simulink model "baseline_auto_parcel_loading_process"  (R2026a)
settings: Solver=VariableStepAuto  StopTime=500  MaxStep=0.05
libraries: sim3dlib x36
(part 1 of 5)
settings Model: PacingRate=1000  Creator=minho  LastModifiedBy=minho

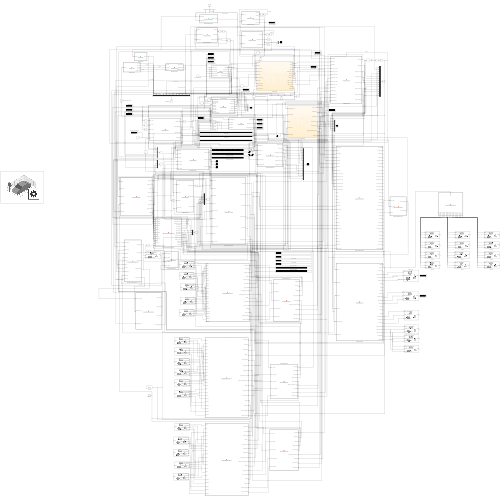
[thumbnail: Simulink's stored preview of the top-level diagram]
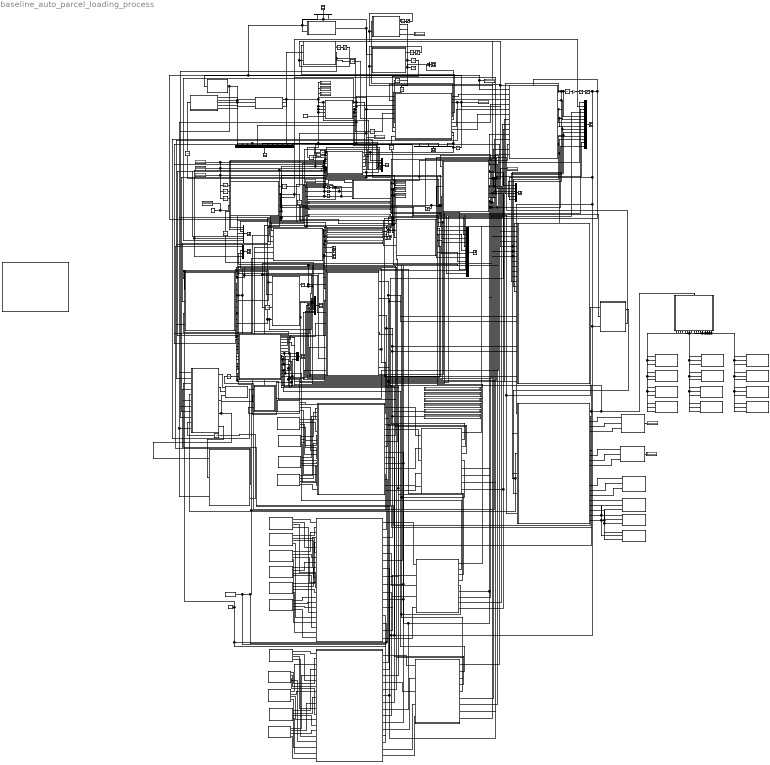
== system baseline_auto_parcel_loading_process ==
  note: floor1_remaining_length
  ArriveDoneDelayToMainController : UnitDelay  SampleTime=0.05
  Belt1_F1 : sim3dlib/Simulation 3D Actor  Priority=1  ActorName=Belt1_F1_Actor  ParentName=Scene Origin  Operation=Create at setup  InitScriptText=|  SampleTime=-1  Translation=[0 0 0]  Rotation=[0 0 0]  Scale=[1 1 1]  InputsText=|  aMode=5  ActorTag=Belt1_F1_Actor  ActorType=Sim3dActor  ID=C
      InitScriptText=|
      | % Reserved keywords:
      | % - Actor : handle to this actor object
      | % - World : handle to the world object
      | 
      | % Examples:
      | 
      | % Create a primitive geometry (optional)
      | createShape(Actor, 'box', [1 1 1]);
      | 
      | % Initialize values (optional)
      | % Actor.Physics = true;
      | Actor.Color = [0.1 0.1 0.1];
      InputsText=|
      | Belt1_F1_Actor.Translation
      | Belt1_F1_Actor.Rotation   
      | Belt1_F1_Actor.Scale
  Belt1_F2 : sim3dlib/Simulation 3D Actor  Priority=1  ActorName=Belt1_F2_Actor  ParentName=Scene Origin  Operation=Create at setup  InitScriptText=|  SampleTime=-1  Translation=[0 0 0]  Rotation=[0 0 0]  Scale=[1 1 1]  InputsText=|  aMode=5  ActorTag=Belt1_F2_Actor  ActorType=Sim3dActor  ID=C
      InitScriptText=|
      | % Reserved keywords:
      | % - Actor : handle to this actor object
      | % - World : handle to the world object
      | createShape(Actor, 'box', [1 1 1]);
      | Actor.Color = [0.1 0.1 0.1];
      | % Examples:
      | 
      | % Create a primitive geometry (optional)
      | % createShape(Actor, 'box', [1 1 1]);
      | 
      | % Initialize values (optional)
      | % Actor.Physics = true;
      | % Actor.Color = [1 0 0];
      InputsText=|
      | Belt1_F2_Actor.Translation
      | Belt1_F2_Actor.Rotation   
      | Belt1_F2_Actor.Scale
  Belt1_F3 : sim3dlib/Simulation 3D Actor  Priority=1  ActorName=Belt1_F3_Actor  ParentName=Scene Origin  Operation=Create at setup  InitScriptText=|  SampleTime=-1  Translation=[0 0 0]  Rotation=[0 0 0]  Scale=[1 1 1]  InputsText=|  aMode=5  ActorTag=Belt1_F3_Actor  ActorType=Sim3dActor  ID=C
      InitScriptText=|
      | % Reserved keywords:
      | % - Actor : handle to this actor object
      | % - World : handle to the world object
      | createShape(Actor, 'box', [1 1 1]);
      | Actor.Color = [0.1 0.1 0.1];
      | % Examples:
      | 
      | % Create a primitive geometry (optional)
      | % createShape(Actor, 'box', [1 1 1]);
      | 
      | % Initialize values (optional)
      | % Actor.Physics = true;
      | % Actor.Color = [1 0 0];
      InputsText=|
      | Belt1_F3_Actor.Translation
      | Belt1_F3_Actor.Rotation   
      | Belt1_F3_Actor.Scale
  Belt2_F1 : sim3dlib/Simulation 3D Actor  Priority=1  ActorName=Belt2_F1_Actor  ParentName=Scene Origin  Operation=Create at setup  InitScriptText=|  SampleTime=-1  Translation=[0 0 0]  Rotation=[0 0 0]  Scale=[1 1 1]  InputsText=|  aMode=5  ActorTag=Belt2_F1_Actor  ActorType=Sim3dActor  ID=C
      InitScriptText=|
      | % Reserved keywords:
      | % - Actor : handle to this actor object
      | % - World : handle to the world object
      | 
      | % Examples:
      | 
      | % Create a primitive geometry (optional)
      | createShape(Actor, 'box', [1 1 1]);
      | 
      | % Initialize values (optional)
      | % Actor.Physics = true;
      | Actor.Color = [0.2 0.2 0.2];
      InputsText=|
      | Belt2_F1_Actor.Translation
      | Belt2_F1_Actor.Rotation   
      | Belt2_F1_Actor.Scale
  Belt2_F2 : sim3dlib/Simulation 3D Actor  Priority=1  ActorName=Belt2_F2_Actor  ParentName=Scene Origin  Operation=Create at setup  InitScriptText=|  SampleTime=-1  Translation=[0 0 0]  Rotation=[0 0 0]  Scale=[1 1 1]  InputsText=|  aMode=5  ActorTag=Belt2_F2_Actor  ActorType=Sim3dActor  ID=C
      InitScriptText=|
      | % Reserved keywords:
      | % - Actor : handle to this actor object
      | % - World : handle to the world object
      | createShape(Actor, 'box', [1 1 1]);
      | Actor.Color = [0.2 0.2 0.2];
      | % Examples:
      | 
      | % Create a primitive geometry (optional)
      | % createShape(Actor, 'box', [1 1 1]);
      | 
      | % Initialize values (optional)
      | % Actor.Physics = true;
      | % Actor.Color = [1 0 0];
      InputsText=|
      | Belt2_F2_Actor.Translation
      | Belt2_F2_Actor.Rotation   
      | Belt2_F2_Actor.Scale
  Belt2_F3 : sim3dlib/Simulation 3D Actor  Priority=1  ActorName=Belt2_F3_Actor  ParentName=Scene Origin  Operation=Create at setup  InitScriptText=|  SampleTime=-1  Translation=[0 0 0]  Rotation=[0 0 0]  Scale=[1 1 1]  InputsText=|  aMode=5  ActorTag=Belt2_F3_Actor  ActorType=Sim3dActor  ID=C
      InitScriptText=|
      | % Reserved keywords:
      | % - Actor : handle to this actor object
      | % - World : handle to the world object
      | createShape(Actor, 'box', [1 1 1]);
      | Actor.Color = [0.2 0.2 0.2];
      | % Examples:
      | 
      | % Create a primitive geometry (optional)
      | % createShape(Actor, 'box', [1 1 1]);
      | 
      | % Initialize values (optional)
      | % Actor.Physics = true;
      | % Actor.Color = [1 0 0];
      InputsText=|
      | Belt2_F3_Actor.Translation
      | Belt2_F3_Actor.Rotation   
      | Belt2_F3_Actor.Scale
  Belt3_F1 : sim3dlib/Simulation 3D Actor  Priority=1  ActorName=Belt3_F1_Actor  ParentName=Scene Origin  Operation=Create at setup  InitScriptText=|  SampleTime=-1  Translation=[0 0 0]  Rotation=[0 0 0]  Scale=[1 1 1]  InputsText=|  aMode=5  ActorTag=Belt3_F1_Actor  ActorType=Sim3dActor  ID=C
      InitScriptText=|
      | % Reserved keywords:
      | % - Actor : handle to this actor object
      | % - World : handle to the world object
      | 
      | % Examples:
      | 
      | % Create a primitive geometry (optional)
      | createShape(Actor, 'box', [1 1 1]);
      | 
      | % Initialize values (optional)
      | % Actor.Physics = true;
      | Actor.Color = [0.3 0.3 0.3];
      InputsText=|
      | Belt3_F1_Actor.Translation
      | Belt3_F1_Actor.Rotation   
      | Belt3_F1_Actor.Scale
  Belt3_F2 : sim3dlib/Simulation 3D Actor  Priority=1  ActorName=Belt3_F2_Actor  ParentName=Scene Origin  Operation=Create at setup  InitScriptText=|  SampleTime=-1  Translation=[0 0 0]  Rotation=[0 0 0]  Scale=[1 1 1]  InputsText=|  aMode=5  ActorTag=Belt3_F2_Actor  ActorType=Sim3dActor  ID=C
      InitScriptText=|
      | % Reserved keywords:
      | % - Actor : handle to this actor object
      | % - World : handle to the world object
      | 
      | % Examples:
      | createShape(Actor, 'box', [1 1 1]);
      | Actor.Color = [0.3 0.3 0.3];
      | % Create a primitive geometry (optional)
      | % createShape(Actor, 'box', [1 1 1]);
      | 
      | % Initialize values (optional)
      | % Actor.Physics = true;
      | % Actor.Color = [1 0 0];
      InputsText=|
      | Belt3_F2_Actor.Translation
      | Belt3_F2_Actor.Rotation   
      | Belt3_F2_Actor.Scale
  Belt3_F3 : sim3dlib/Simulation 3D Actor  Priority=1  ActorName=Belt3_F3_Actor  ParentName=Scene Origin  Operation=Create at setup  InitScriptText=|  SampleTime=-1  Translation=[0 0 0]  Rotation=[0 0 0]  Scale=[1 1 1]  InputsText=|  aMode=5  ActorTag=Belt3_F3_Actor  ActorType=Sim3dActor  ID=C
      InitScriptText=|
      | % Reserved keywords:
      | % - Actor : handle to this actor object
      | % - World : handle to the world object
      | createShape(Actor, 'box', [1 1 1]);
      | Actor.Color = [0.3 0.3 0.3];
      | % Examples:
      | 
      | % Create a primitive geometry (optional)
      | % createShape(Actor, 'box', [1 1 1]);
      | 
      | % Initialize values (optional)
      | % Actor.Physics = true;
      | % Actor.Color = [1 0 0];
      InputsText=|
      | Belt3_F3_Actor.Translation
      | Belt3_F3_Actor.Rotation   
      | Belt3_F3_Actor.Scale
  Belt4_F1 : sim3dlib/Simulation 3D Actor  Priority=1  ActorName=Belt4_F1_Actor  ParentName=Scene Origin  Operation=Create at setup  InitScriptText=|  SampleTime=-1  Translation=[0 0 0]  Rotation=[0 0 0]  Scale=[1 1 1]  InputsText=|  aMode=5  ActorTag=Belt4_F1_Actor  ActorType=Sim3dActor  ID=C
      InitScriptText=|
      | % Reserved keywords:
      | % - Actor : handle to this actor object
      | % - World : handle to the world object
      | 
      | % Examples:
      | 
      | % Create a primitive geometry (optional)
      | createShape(Actor, 'box', [1 1 1]);
      | 
      | % Initialize values (optional)
      | % Actor.Physics = true;
      | Actor.Color = [0.4 0.4 0.4];
      InputsText=|
      | Belt4_F1_Actor.Translation
      | Belt4_F1_Actor.Rotation   
      | Belt4_F1_Actor.Scale
  Belt4_F2 : sim3dlib/Simulation 3D Actor  Priority=1  ActorName=Belt4_F2_Actor  ParentName=Scene Origin  Operation=Create at setup  InitScriptText=|  SampleTime=-1  Translation=[0 0 0]  Rotation=[0 0 0]  Scale=[1 1 1]  InputsText=|  aMode=5  ActorTag=Belt4_F2_Actor  ActorType=Sim3dActor  ID=C
      InitScriptText=|
      | % Reserved keywords:
      | % - Actor : handle to this actor object
      | % - World : handle to the world object
      | createShape(Actor, 'box', [1 1 1]);
      | Actor.Color = [0.4 0.4 0.4];
      | % Examples:
      | 
      | % Create a primitive geometry (optional)
      | % createShape(Actor, 'box', [1 1 1]);
      | 
      | % Initialize values (optional)
      | % Actor.Physics = true;
      | % Actor.Color = [1 0 0];
      InputsText=|
      | Belt4_F2_Actor.Translation
      | Belt4_F2_Actor.Rotation   
      | Belt4_F2_Actor.Scale
  Belt4_F3 : sim3dlib/Simulation 3D Actor  Priority=1  ActorName=Belt4_F3_Actor  ParentName=Scene Origin  Operation=Create at setup  InitScriptText=|  SampleTime=-1  Translation=[0 0 0]  Rotation=[0 0 0]  Scale=[1 1 1]  InputsText=|  aMode=5  ActorTag=Belt4_F3_Actor  ActorType=Sim3dActor  ID=C
      InitScriptText=|
      | % Reserved keywords:
      | % - Actor : handle to this actor object
      | % - World : handle to the world object
      | createShape(Actor, 'box', [1 1 1]);
      | Actor.Color = [0.4 0.4 0.4];
      | % Examples:
      | 
      | % Create a primitive geometry (optional)
      | % createShape(Actor, 'box', [1 1 1]);
      | 
      | % Initialize values (optional)
      | % Actor.Physics = true;
      | % Actor.Color = [1 0 0];
      InputsText=|
      | Belt4_F3_Actor.Translation
      | Belt4_F3_Actor.Rotation   
      | Belt4_F3_Actor.Scale
  BoxPoseFunction : MATLAB Function  TreatAsAtomicUnit=on
  BoxRotationFunction : MATLAB Function  TreatAsAtomicUnit=on
  BoxSizeFunction : MATLAB Function  TreatAsAtomicUnit=on
  CommandMuxFunction : MATLAB Function  TreatAsAtomicUnit=on
  Conveyor3DMappingFunction : MATLAB Function  TreatAsAtomicUnit=on
  CurrentUnloadReadySelector : MATLAB Function  TreatAsAtomicUnit=on
  Delay_current_target_package_id : UnitDelay  SampleTime=0.05
  Delay_floor1_queue : UnitDelay  InitialCondition=zeros(50,1)  SampleTime=-1
  Delay_floor2_queue : UnitDelay  InitialCondition=zeros(50,1)  SampleTime=-1
  Delay_floor3_queue : UnitDelay  InitialCondition=zeros(50,1)  SampleTime=-1
  Delay_load_done_for_box : UnitDelay  SampleTime=-1
  Delay_unload_all_done_to_mission : UnitDelay  SampleTime=-1
  Delay_unload_done_to_target_manager : UnitDelay  SampleTime=0.05
  Display : Display
  Display1 : Display
  Floor1VisualStateFunction : MATLAB Function  TreatAsAtomicUnit=on
  Floor2VisualStateFunction : MATLAB Function  TreatAsAtomicUnit=on  SystemSampleTime=0.05
  Floor3VisualStateFunction : MATLAB Function  TreatAsAtomicUnit=on  SystemSampleTime=0.05
  FloorStorageUpdate : MATLAB Function  TreatAsAtomicUnit=on
  FloorUnloadTargetSelector : MATLAB Function  TreatAsAtomicUnit=on
  Gain : Gain  Gain=0.075
  Integrator{,1..3} (4 alike) : Integrator
  MATLAB Function : MATLAB Function  TreatAsAtomicUnit=on
  MATLAB Function1 : MATLAB Function  TreatAsAtomicUnit=on
  MATLAB Function3 : MATLAB Function  TreatAsAtomicUnit=on  SystemSampleTime=0.05
  MainController : Stateflow chart  TreatAsAtomicUnit=on
  MissionModeFunction : MATLAB Function  TreatAsAtomicUnit=on  SystemSampleTime=0.05
  MovingPackage3DMappingFunction : MATLAB Function  TreatAsAtomicUnit=on  SystemSampleTime=0.05
  MultiFloorUnloadPrepositionFunction : MATLAB Function  TreatAsAtomicUnit=on  SystemSampleTime=0.05
  Mux : Mux  Inputs=12
  Mux1 : Mux  Inputs=6
  Mux10 : Mux  Inputs=3
  Mux17 : Mux  Inputs=9
  Mux2 : Mux  Inputs=12
  Mux3 : Mux
  Mux4 : Mux  Inputs=13
  Mux5 : Mux  Inputs=14
  Mux6 : Mux  Inputs=7
  Mux7 : Mux
  Mux8 : Mux  Inputs=3
  Mux9 : Mux  Inputs=3
  Package3DMappingFunction_F2 : MATLAB Function  TreatAsAtomicUnit=on
  PackageSlotToXYZFunction : MATLAB Function  TreatAsAtomicUnit=on
  PackageSlotVisualizer : MATLAB Function  TreatAsAtomicUnit=on
  PlatformFoldControlFunction : MATLAB Function  TreatAsAtomicUnit=on  SystemSampleTime=0.05
  Platform_Actor : sim3dlib/Simulation 3D Actor  Priority=1  ActorName=Platform_Actor  ParentName=Scene Origin  Operation=Create at setup  InitScriptText=|  SampleTime=-1  Translation=[0 0 0]  Rotation=[0 0 0]  Scale=[1 1 1]  InputsText=|  aMode=5  ActorTag=Platform_Actor  ActorType=Sim3dActor  ID=C
      InitScriptText=|
      | % Reserved keywords:
      | % - Actor : handle to this actor object
      | % - World : handle to the world object
      | 
      | % Examples:
      | 
      | % Create a primitive geometry (optional)
      | createShape(Actor, 'box', [0.25 0.25 0.04]);
      | 
      | % Initialize values (optional)
      | % Actor.Physics = true;
      | % Actor.Color = [1 0 0];
      InputsText=|
      | Platform_Actor.Translation
      | Platform_Actor.Rotation   
      | Platform_Actor.Scale
  PusherControlFunction : MATLAB Function  TreatAsAtomicUnit=on  SystemSampleTime=0.05
  RotatorControlFunction : MATLAB Function  TreatAsAtomicUnit=on
  Saturation : Saturate  UpperLimit=90  LowerLimit=-90
  Saturation1 : Saturate  UpperLimit=0.54  LowerLimit=0
  Saturation2 : Saturate  UpperLimit=0.24  LowerLimit=0
  Saturation3 : Saturate  UpperLimit=1  LowerLimit=0
  Scope{,2..12} (12 alike) : Scope
      Scope settings: ActiveDisplayYMinimum=-0.20375306954883365  ActiveDisplayYMaximum=1.6708362727347574  DataLoggingVariableName=ScopeData3
      Scope10 settings: DataLoggingVariableName=ScopeData11
      Scope11 settings: DataLoggingVariableName=ScopeData12
      Scope12 settings: DataLoggingVariableName=ScopeData13
      Scope2 settings: ActiveDisplayYMinimum=-2.7964097544610729  ActiveDisplayYMaximum=6.6483838032738971
      Scope3 settings: ActiveDisplayYMinimum=-5.3367793063666333  ActiveDisplayYMaximum=11.034780106497895
      Scope4 settings: ActiveDisplayYMinimum=-0.99999999999999978  ActiveDisplayYMaximum=9  DataLoggingVariableName=ScopeData4
      Scope5 settings: ActiveDisplayYMinimum=0.14637662084101377  ActiveDisplayYMaximum=19.945692615235014  DataLoggingVariableName=ScopeData5
      Scope6 settings: ActiveDisplayYMinimum=-0.24999999999999994  ActiveDisplayYMaximum=2.25  DataLoggingVariableName=ScopeData19
      Scope7 settings: ActiveDisplayYMinimum=-1  ActiveDisplayYMaximum=1  DataLoggingVariableName=ScopeData6
      Scope8 settings: DataLoggingVariableName=ScopeData7
      Scope9 settings: ActiveDisplayYMinimum=-3.52364966859015  ActiveDisplayYMaximum=17.689903182546253  DataLoggingVariableName=ScopeData8
  Sim3DMappingFunction : MATLAB Function  TreatAsAtomicUnit=on
  Simulation 3D Actor : sim3dlib/Simulation 3D Actor  Priority=1  ActorName=Rotator_Actor  ParentName=Scene Origin  Operation=Create at setup  InitScriptText=|  SampleTime=-1  Translation=[0 0 0]  Rotation=[0 0 0]  Scale=[1 1 1]  InputsText=|  aMode=5  ActorTag=Rotator_Actor  ActorType=Sim3dActor  ID=C
      InitScriptText=|
      | % Reserved keywords:
      | % - Actor : handle to this actor object
      | % - World : handle to the world object
      | 
      | % Examples:
      | 
      | % Create a primitive geometry (optional)
      | createShape(Actor, 'cylinder', [0.20 0.20 0.001]);
      | 
      | % Initialize values (optional)
      | % Actor.Physics = true;
      | Actor.Color = [1 0 0];
      InputsText=|
      | Rotator_Actor.Translation
      | Rotator_Actor.Rotation   
      | Rotator_Actor.Scale
  Simulation 3D Actor1 : sim3dlib/Simulation 3D Actor  Priority=1  ActorName=Pusher_Actor  ParentName=Scene Origin  Operation=Create at setup  InitScriptText=|  SampleTime=-1  Translation=[0 0 0]  Rotation=[0 0 0]  Scale=[1 1 1]  InputsText=|  aMode=5  ActorTag=Pusher_Actor  ActorType=Sim3dActor  ID=C
      InitScriptText=|
      | % Reserved keywords:
      | % - Actor : handle to this actor object
      | % - World : handle to the world object
      | 
      | % Examples:
      | 
      | % Create a primitive geometry (optional)
      | createShape(Actor, 'box', [0.20 0.03 0.04]);
      | 
      | % Initialize values (optional)
      | % Actor.Physics = true;
      | Actor.Color = [0 1 0];
      InputsText=|
      | Pusher_Actor.Translation
      | Pusher_Actor.Rotation   
      | Pusher_Actor.Scale
  Simulation 3D Actor10 : sim3dlib/Simulation 3D Actor  Priority=1  ActorName=MovingPackage_Actor  ParentName=Scene Origin  Operation=Create at setup  InitScriptText=|  SampleTime=-1  Translation=[0 0 0]  Rotation=[0 0 0]  Scale=[1 1 1]  InputsText=|  aMode=5  ActorTag=MovingPackage_Actor  ActorType=Sim3dActor  ID=C
      | createShape(Actor, 'box', [1 1 1]);
      | Actor.Color = [0.75 0.45 0.20];
      | % Examples:
      | 
      | % Create a primitive geometry (optional)
      | % createShape(Actor, 'box', [1 1 1]);
      | 
      | % Initialize values (optional)
      | % Actor.Physics = true;
      | % Actor.Color = [1 0 0];
      | MovingPackage_Actor.Translation
      | MovingPackage_Actor.Rotation   
      | MovingPackage_Actor.Scale
  Simulation 3D Actor11 : sim3dlib/Simulation 3D Actor  Priority=1  ActorName=Package1_1_Actor  ParentName=Scene Origin  Operation=Create at setup  InitScriptText=|  SampleTime=-1  Translation=[0 0 0]  Rotation=[0 0 0]  Scale=[1 1 1]  InputsText=|  aMode=5  ActorTag=Package1_1_Actor  ActorType=Sim3dActor  ID=C
      InitScriptText=|
      | % Reserved keywords:
      | % - Actor : handle to this actor object
      | % - World : handle to the world object
      | createShape(Actor, 'box', [1 1 1]);
      | Actor.Color = [0.75 0.45 0.20];
      | % Examples:
      | 
      | % Create a primitive geometry (optional)
      | % createShape(Actor, 'box', [1 1 1]);
      | 
      | % Initialize values (optional)
      | % Actor.Physics = true;
      | % Actor.Color = [1 0 0];
      InputsText=|
      | Package1_1_Actor.Translation
      | Package1_1_Actor.Rotation   
      | Package1_1_Actor.Scale      
      | Package1_1_Actor.Color
  Simulation 3D Actor12 : sim3dlib/Simulation 3D Actor  Priority=1  ActorName=Package1_4_Actor  ParentName=Scene Origin  Operation=Create at setup  InitScriptText=|  SampleTime=-1  Translation=[0 0 0]  Rotation=[0 0 0]  Scale=[1 1 1]  InputsText=|  aMode=5  ActorTag=Package1_4_Actor  ActorType=Sim3dActor  ID=C
      InitScriptText=|
      | % Reserved keywords:
      | % - Actor : handle to this actor object
      | % - World : handle to the world object
      | createShape(Actor, 'box', [1 1 1]);
      | Actor.Color = [0.75 0.45 0.20];
      | % Examples:
      | 
      | % Create a primitive geometry (optional)
      | % createShape(Actor, 'box', [1 1 1]);
      | 
      | % Initialize values (optional)
      | % Actor.Physics = true;
      | % Actor.Color = [1 0 0];
      InputsText=|
      | Package1_4_Actor.Translation
      | Package1_4_Actor.Rotation   
      | Package1_4_Actor.Scale      
      | Package1_4_Actor.Color
  Simulation 3D Actor13 : sim3dlib/Simulation 3D Actor  Priority=1  ActorName=Package1_5_Actor  ParentName=Scene Origin  Operation=Create at setup  InitScriptText=|  SampleTime=-1  Translation=[0 0 0]  Rotation=[0 0 0]  Scale=[1 1 1]  InputsText=|  aMode=5  ActorTag=Package1_5_Actor  ActorType=Sim3dActor  ID=C
      InitScriptText=|
      | % Reserved keywords:
      | % - Actor : handle to this actor object
      | % - World : handle to the world object
      | createShape(Actor, 'box', [1 1 1]);
      | Actor.Color = [0.75 0.45 0.20];
      | % Examples:
      | 
      | % Create a primitive geometry (optional)
      | % createShape(Actor, 'box', [1 1 1]);
      | 
      | % Initialize values (optional)
      | % Actor.Physics = true;
      | % Actor.Color = [1 0 0];
      InputsText=|
      | Package1_5_Actor.Translation
      | Package1_5_Actor.Rotation   
      | Package1_5_Actor.Scale      
      | Package1_5_Actor.Color
  Simulation 3D Actor14 : sim3dlib/Simulation 3D Actor  Priority=1  ActorName=Package3_1_Actor  ParentName=Scene Origin  Operation=Create at setup  InitScriptText=|  SampleTime=-1  Translation=[0 0 0]  Rotation=[0 0 0]  Scale=[1 1 1]  InputsText=|  aMode=5  ActorTag=Package3_1_Actor  ActorType=Sim3dActor  ID=C
      InitScriptText=|
      | % Reserved keywords:
      | % - Actor : handle to this actor object
      | % - World : handle to the world object
      | createShape(Actor, 'box', [1 1 1]);
      | Actor.Color = [0.75 0.45 0.20];
      | % Examples:
      | 
      | % Create a primitive geometry (optional)
      | % createShape(Actor, 'box', [1 1 1]);
      | 
      | % Initialize values (optional)
      | % Actor.Physics = true;
      | % Actor.Color = [1 0 0];
      InputsText=|
      | Package3_1_Actor.Translation
      | Package3_1_Actor.Rotation   
      | Package3_1_Actor.Scale      
      | Package3_1_Actor.Color
  Simulation 3D Actor15 : sim3dlib/Simulation 3D Actor  Priority=1  ActorName=Package3_4_Actor  ParentName=Scene Origin  Operation=Create at setup  InitScriptText=|  SampleTime=-1  Translation=[0 0 0]  Rotation=[0 0 0]  Scale=[1 1 1]  InputsText=|  aMode=5  ActorTag=Package3_4_Actor  ActorType=Sim3dActor  ID=C
      InitScriptText=|
      | % Reserved keywords:
      | % - Actor : handle to this actor object
      | % - World : handle to the world object
      | createShape(Actor, 'box', [1 1 1]);
      | Actor.Color = [0.75 0.45 0.20];
      | % Examples:
      | 
      | % Create a primitive geometry (optional)
      | % createShape(Actor, 'box', [1 1 1]);
      | 
      | % Initialize values (optional)
      | % Actor.Physics = true;
      | % Actor.Color = [1 0 0];
      InputsText=|
      | Package3_4_Actor.Translation
      | Package3_4_Actor.Rotation   
      | Package3_4_Actor.Scale      
      | Package3_4_Actor.Color
  Simulation 3D Actor16 : sim3dlib/Simulation 3D Actor  Priority=1  ActorName=Package3_5_Actor  ParentName=Scene Origin  Operation=Create at setup  InitScriptText=|  SampleTime=-1  Translation=[0 0 0]  Rotation=[0 0 0]  Scale=[1 1 1]  InputsText=|  aMode=5  ActorTag=Package3_5_Actor  ActorType=Sim3dActor  ID=C
      InitScriptText=|
      | % Reserved keywords:
      | % - Actor : handle to this actor object
      | % - World : handle to the world object
      | createShape(Actor, 'box', [1 1 1]);
      | Actor.Color = [0.75 0.45 0.20];
      | % Examples:
      | 
      | % Create a primitive geometry (optional)
      | % createShape(Actor, 'box', [1 1 1]);
      | 
      | % Initialize values (optional)
      | % Actor.Physics = true;
      | % Actor.Color = [1 0 0];
      InputsText=|
      | Package3_5_Actor.Translation
      | Package3_5_Actor.Rotation   
      | Package3_5_Actor.Scale      
      | Package3_5_Actor.Color
  Simulation 3D Actor17 : sim3dlib/Simulation 3D Actor  Priority=1  ActorName=Package1_2_Actor  ParentName=Scene Origin  Operation=Create at setup  InitScriptText=|  SampleTime=-1  Translation=[0 0 0]  Rotation=[0 0 0]  Scale=[1 1 1]  InputsText=|  aMode=5  ActorTag=Package1_2_Actor  ActorType=Sim3dActor  ID=C
      InitScriptText=|
      | % Reserved keywords:
      | % - Actor : handle to this actor object
      | % - World : handle to the world object
      | createShape(Actor, 'box', [1 1 1]);
      | Actor.Color = [0.75 0.45 0.20];
      | % Examples:
      | 
      | % Create a primitive geometry (optional)
      | % createShape(Actor, 'box', [1 1 1]);
      | 
      | % Initialize values (optional)
      | % Actor.Physics = true;
      | % Actor.Color = [1 0 0];
      InputsText=|
      | Package1_2_Actor.Translation
      | Package1_2_Actor.Rotation   
      | Package1_2_Actor.Scale      
      | Package1_2_Actor.Color
  Simulation 3D Actor18 : sim3dlib/Simulation 3D Actor  Priority=1  ActorName=Package1_3_Actor  ParentName=Scene Origin  Operation=Create at setup  InitScriptText=|  SampleTime=-1  Translation=[0 0 0]  Rotation=[0 0 0]  Scale=[1 1 1]  InputsText=|  aMode=5  ActorTag=Package1_3_Actor  ActorType=Sim3dActor  ID=C
      InitScriptText=|
      | % Reserved keywords:
      | % - Actor : handle to this actor object
      | % - World : handle to the world object
      | createShape(Actor, 'box', [1 1 1]);
      | Actor.Color = [0.75 0.45 0.20];
      | % Examples:
      | 
      | % Create a primitive geometry (optional)
      | % createShape(Actor, 'box', [1 1 1]);
      | 
      | % Initialize values (optional)
      | % Actor.Physics = true;
      | % Actor.Color = [1 0 0];
      InputsText=|
      | Package1_3_Actor.Translation
      | Package1_3_Actor.Rotation   
      | Package1_3_Actor.Scale      
      | Package1_3_Actor.Color
  Simulation 3D Actor19 : sim3dlib/Simulation 3D Actor  Priority=1  ActorName=Package3_3_Actor  ParentName=Scene Origin  Operation=Create at setup  InitScriptText=|  SampleTime=-1  Translation=[0 0 0]  Rotation=[0 0 0]  Scale=[1 1 1]  InputsText=|  aMode=5  ActorTag=Package3_3_Actor  ActorType=Sim3dActor  ID=C
      InitScriptText=|
      | % Reserved keywords:
      | % - Actor : handle to this actor object
      | % - World : handle to the world object
      | createShape(Actor, 'box', [1 1 1]);
      | Actor.Color = [0.75 0.45 0.20];
      | % Examples:
      | 
      | % Create a primitive geometry (optional)
      | % createShape(Actor, 'box', [1 1 1]);
      | 
      | % Initialize values (optional)
      | % Actor.Physics = true;
      | % Actor.Color = [1 0 0];
      InputsText=|
      | Package3_3_Actor.Translation
      | Package3_3_Actor.Rotation   
      | Package3_3_Actor.Scale      
      | Package3_3_Actor.Color
  Simulation 3D Actor2 : sim3dlib/Simulation 3D Actor  Priority=1  ActorName=Stopper_F1_Actor  ParentName=Scene Origin  Operation=Create at setup  InitScriptText=|  SampleTime=-1  Translation=[0 0 0]  Rotation=[0 0 0]  Scale=[1 1 1]  InputsText=|  aMode=5  ActorTag=Stopper_F1_Actor  ActorType=Sim3dActor  ID=C
      InitScriptText=|
      | % Reserved keywords:
      | % - Actor : handle to this actor object
      | % - World : handle to the world object
      | 
      | % Examples:
      | 
      | % Create a primitive geometry (optional)
      | createShape(Actor, 'box', [0.03 0.25 0.10]);
      | 
      | % Initialize values (optional)
      | % Actor.Physics = true;
      | Actor.Color = [1 1 0];
      InputsText=|
      | Stopper_F1_Actor.Translation
      | Stopper_F1_Actor.Rotation   
      | Stopper_F1_Actor.Scale
  Simulation 3D Actor20 : sim3dlib/Simulation 3D Actor  Priority=1  ActorName=Package3_2_Actor  ParentName=Scene Origin  Operation=Create at setup  InitScriptText=|  SampleTime=-1  Translation=[0 0 0]  Rotation=[0 0 0]  Scale=[1 1 1]  InputsText=|  aMode=5  ActorTag=Package3_2_Actor  ActorType=Sim3dActor  ID=C
      InitScriptText=|
      | % Reserved keywords:
      | % - Actor : handle to this actor object
      | % - World : handle to the world object
      | createShape(Actor, 'box', [1 1 1]);
      | Actor.Color = [0.75 0.45 0.20];
      | % Examples:
      | 
      | % Create a primitive geometry (optional)
      | % createShape(Actor, 'box', [1 1 1]);
      | 
      | % Initialize values (optional)
      | % Actor.Physics = true;
      | % Actor.Color = [1 0 0];
      InputsText=|
      | Package3_2_Actor.Translation
      | Package3_2_Actor.Rotation   
      | Package3_2_Actor.Scale      
      | Package3_2_Actor.Color
  Simulation 3D Actor21 : sim3dlib/Simulation 3D Actor  Priority=1  ActorName=Package2_6_Actor  ParentName=Scene Origin  Operation=Create at setup  InitScriptText=|  SampleTime=-1  Translation=[0 0 0]  Rotation=[0 0 0]  Scale=[1 1 1]  InputsText=|  aMode=5  ActorTag=Package2_6_Actor  ActorType=Sim3dActor  ID=C
      InitScriptText=|
      | % Reserved keywords:
      | % - Actor : handle to this actor object
      | % - World : handle to the world object
      | 
      | % Examples:
      | 
      | % Create a primitive geometry (optional)
      | createShape(Actor, 'box', [1 1 1]);
      | Actor.Color = [0.75 0.45 0.20];
      | 
      | % Initialize values (optional)
      | % Actor.Physics = true;
      InputsText=|
      | Package2_6_Actor.Translation
      | Package2_6_Actor.Rotation   
      | Package2_6_Actor.Scale      
      | Package2_6_Actor.Color
  Simulation 3D Actor3 : sim3dlib/Simulation 3D Actor  Priority=1  ActorName=Stopper_F3_Actor  ParentName=Scene Origin  Operation=Create at setup  InitScriptText=|  SampleTime=-1  Translation=[0 0 0]  Rotation=[0 0 0]  Scale=[1 1 1]  InputsText=|  aMode=5  ActorTag=Stopper_F3_Actor  ActorType=Sim3dActor  ID=C
      InitScriptText=|
      | % Reserved keywords:
      | % - Actor : handle to this actor object
      | % - World : handle to the world object
      | 
      | % Examples:
      | 
      | % Create a primitive geometry (optional)
      | createShape(Actor, 'box', [0.03 0.25 0.10]);
      | 
      | % Initialize values (optional)
      | % Actor.Physics = true;
      | Actor.Color = [1 1 0];
      InputsText=|
      | Stopper_F3_Actor.Translation
      | Stopper_F3_Actor.Rotation   
      | Stopper_F3_Actor.Scale
  Simulation 3D Actor4 : sim3dlib/Simulation 3D Actor  Priority=1  ActorName=Stopper_F2_Actor  ParentName=Scene Origin  Operation=Create at setup  InitScriptText=|  SampleTime=-1  Translation=[0 0 0]  Rotation=[0 0 0]  Scale=[1 1 1]  InputsText=|  aMode=5  ActorTag=Stopper_F2_Actor  ActorType=Sim3dActor  ID=C
      InitScriptText=|
      | % Reserved keywords:
      | % - Actor : handle to this actor object
      | % - World : handle to the world object
      | 
      | % Examples:
      | 
      | % Create a primitive geometry (optional)
      | createShape(Actor, 'box', [0.03 0.25 0.10]);
      | 
      | % Initialize values (optional)
      | % Actor.Physics = true;
      | Actor.Color = [1 1 0];
      InputsText=|
      | Stopper_F2_Actor.Translation
      | Stopper_F2_Actor.Rotation   
      | Stopper_F2_Actor.Scale
  Simulation 3D Actor5 : sim3dlib/Simulation 3D Actor  Priority=1  ActorName=Package2_1_Actor  ParentName=Scene Origin  Operation=Create at setup  InitScriptText=|  SampleTime=-1  Translation=[0 0 0]  Rotation=[0 0 0]  Scale=[1 1 1]  InputsText=|  aMode=5  ActorTag=Package2_1_Actor  ActorType=Sim3dActor  ID=C
      | createShape(Actor, 'box', [1 1 1]);
      | Actor.Color = [0.75 0.45 0.20];
      | % Create a primitive geometry (optional)
      | % createShape(Actor, 'box', [1 1 1]);
      | 
      | % Initialize values (optional)
      | % Actor.Physics = true;
      | % Actor.Color = [1 0 0];
      | Package2_1_Actor.Translation
      | Package2_1_Actor.Rotation   
      | Package2_1_Actor.Scale      
      | Package2_1_Actor.Color
  Simulation 3D Actor6 : sim3dlib/Simulation 3D Actor  Priority=1  ActorName=Package2_2_Actor  ParentName=Scene Origin  Operation=Create at setup  InitScriptText=|  SampleTime=-1  Translation=[0 0 0]  Rotation=[0 0 0]  Scale=[1 1 1]  InputsText=|  aMode=5  ActorTag=Package2_2_Actor  ActorType=Sim3dActor  ID=C
      | createShape(Actor, 'box', [1 1 1]);
      | Actor.Color = [0.75 0.45 0.20];
      | % Examples:
      | 
      | % Create a primitive geometry (optional)
      | % createShape(Actor, 'box', [1 1 1]);
      | 
      | % Initialize values (optional)
      | % Actor.Physics = true;
      | % Actor.Color = [1 0 0];
      | Package2_2_Actor.Translation
      | Package2_2_Actor.Rotation   
      | Package2_2_Actor.Scale      
      | Package2_2_Actor.Color
  Simulation 3D Actor7 : sim3dlib/Simulation 3D Actor  Priority=1  ActorName=Package2_3_Actor  ParentName=Scene Origin  Operation=Create at setup  InitScriptText=|  SampleTime=-1  Translation=[0 0 0]  Rotation=[0 0 0]  Scale=[1 1 1]  InputsText=|  aMode=5  ActorTag=Package2_3_Actor  ActorType=Sim3dActor  ID=C
      | createShape(Actor, 'box', [1 1 1]);
      | Actor.Color = [0.75 0.45 0.20];
      | 
      | % Create a primitive geometry (optional)
      | % createShape(Actor, 'box', [1 1 1]);
      | 
      | % Initialize values (optional)
      | % Actor.Physics = true;
      | % Actor.Color = [1 0 0];
      | Package2_3_Actor.Translation
      | Package2_3_Actor.Rotation   
      | Package2_3_Actor.Scale      
      | Package2_3_Actor.Color
  Simulation 3D Actor8 : sim3dlib/Simulation 3D Actor  Priority=1  ActorName=Package2_4_Actor  ParentName=Scene Origin  Operation=Create at setup  InitScriptText=|  SampleTime=-1  Translation=[0 0 0]  Rotation=[0 0 0]  Scale=[1 1 1]  InputsText=|  aMode=5  ActorTag=Package2_4_Actor  ActorType=Sim3dActor  ID=C
      | createShape(Actor, 'box', [1 1 1]);
      | Actor.Color = [0.75 0.45 0.20];
      | % Examples:
      | 
      | % Create a primitive geometry (optional)
      | % createShape(Actor, 'box', [1 1 1]);
      | 
      | % Initialize values (optional)
      | % Actor.Physics = true;
      | % Actor.Color = [1 0 0];
      | Package2_4_Actor.Translation
      | Package2_4_Actor.Rotation   
      | Package2_4_Actor.Scale      
      | Package2_4_Actor.Color
  Simulation 3D Actor9 : sim3dlib/Simulation 3D Actor  Priority=1  ActorName=Package2_5_Actor  ParentName=Scene Origin  Operation=Create at setup  InitScriptText=|  SampleTime=-1  Translation=[0 0 0]  Rotation=[0 0 0]  Scale=[1 1 1]  InputsText=|  aMode=5  ActorTag=Package2_5_Actor  ActorType=Sim3dActor  ID=C
      | createShape(Actor, 'box', [1 1 1]);
      | Actor.Color = [0.75 0.45 0.20];
      | % Examples:
      | 
      | % Create a primitive geometry (optional)
      | % createShape(Actor, 'box', [1 1 1]);
      | 
      | % Initialize values (optional)
      | % Actor.Physics = true;
      | % Actor.Color = [1 0 0];
      | Package2_5_Actor.Translation
      | Package2_5_Actor.Rotation   
      | Package2_5_Actor.Scale      
      | Package2_5_Actor.Color
  Simulation 3D Scene Configuration : sim3dlib/Simulation 3D Scene Configuration  Priority=0  ProjectFormat=Default Scenes  SceneDesc=Empty scene  ProjectName=C:\Program Files\MATLAB\R2026a\toolbox\shared\sim3d_projects\automotive_project_windows\UE\WindowsNoEditor\VehicleSimulation.exe  ScenePath=/Game/Maps/HwStrght  EnableOpenDRIVE=off  vehTagList={'Belt1_F1_Actor';'Belt1_F2_Actor';'Belt1_F3_Actor';'Belt2_F1_Actor';'Belt2_F2_Actor';'Belt2_F3_Actor';'Belt3_F1_Actor';'Belt3_F2_Actor';'Belt3_F3_Actor';'Belt4_F1_Actor';'Belt4_F2_Actor';'Belt4_F3_Actor';'Custom';'MovingPackage_Actor';'Package1_1_Actor';'Package1_2_Actor';'Package1_3_Actor';'Package1_4_Actor';'Package1_5_Actor';'Package2_1_Actor';'Package2_2_Actor';'Package2_3_Actor';'Package2_4_Actor';'Package2_5_Actor';'Package2_6_Actor';'Package3_1_Actor';'Package3_2_Actor';'Package3_3_Actor';'Package3_4_Actor';'Package3_5_Actor';'Platform_Actor';'Pusher_Actor';'Rotator_Actor';'Scene Origin';'Stopper_F1_Actor';'Stopper_F2_Actor';'Stopper_F3_Actor'}  vehTag=Scene Origin  AttachedCameraRelativeTranslation=[0 0 0]  FreeCameraDefaultInitialTranslation=[-6, 0, 2]  AttachedCameraRelativeRotation=[0, -15, 0]  FreeCameraDefaultInitialRotation=[0, -15, 0]  ViewpointName=Custom  FreeCameraInitialTranslation=[0, 0, 0]  FreeCameraInitialRotation=[0, 0, 0]  OpVisEn=off  Ts=0.2  EnableWindow=on  EnableRemoteAccess=off  SimulationMode=CoSimulation  SimulateUsing=Interpreted execution  EnableAnimationRecording=off  OverrideDefaultRecording=off  AnimationRecordingFileName=sim3dAnimation.mat  AnimationRecordingInterval=[0 inf]  EnableWeather=off  SunAzimuth=90  SunAltitude=40.0  EnableGeospatialSun=off  Latitude=0  Longitude=0  Date=2023-01-01  Time=10:30:00  GeoTimeZone=-5.0  SunDaylightSaving=off  wind=1  clouds=10  EnableVolumetricClouds=off  CloudCoverage=0  CloudAltitude=6  fog=0  rain=0  RaindropsEffect=off  SnowDensity=0  EnableGeospatial=off  TilesetSource=Earth terrain  UseTrueOrigin=off  OriginHeight=200  OriginLatitude=40.744652  OriginLongitude=-73.988864  MapStyle=Aerial  AdditionalAssetIDs=[]  UseAdvancedSunSky=off  SolarTime=11  TimeZone=-5  Day=21  Month=9  Year=2022  UseDaylightSavingTime=on  DSTStartDay=10  DSTStartMonth=3  DSTEndDay=3  DSTEndMonth=11  DSTSwitchHour=2  sensorTag=MainCamera1  sensorId=1  sensorName=MainCamera1  mountLoc=Origin  offsetFlag=off  tmountOffset=[0, 0, 0]  rmountOffset=[0, 0, 0]  HorizontalResolution=1280  VerticalResolution=720  HorizontalFOV=60  mountPoint=[0 0 0]  mountOrientation=[0 0 0]  aMode=5  ID=1  GeoTrigger=Inactive  ViewNameList={'Custom'}  ViewTranslationList={'[0 0 0]'}  ViewRotationList={'[0 0 0]'}
      settings: LibrarySourceBlock=sl3dlib/Simulation 3D/Environment/Simulation 3D Scene Configuration
  Step : Step  Time=430  SampleTime=0
  Step1 : Step  Time=350  SampleTime=0
  Step2 : Step  Time=390  FinalValue=-1  SampleTime=0
  Step3 : Step  Time=430  SampleTime=0
  StopperCommandFunction : MATLAB Function  TreatAsAtomicUnit=on
  StopperControlFunction : MATLAB Function  TreatAsAtomicUnit=on
  StopperScope : Scope
      settings: ActiveDisplayYMinimum=-0.41799344154282014  ActiveDisplayYMaximum=1.2571261092384307  DataLoggingVariableName=ScopeData9
  StopperScopeFinal : Scope
      settings: ActiveDisplayYMinimum=-2.0791149676193323  ActiveDisplayYMaximum=2.5877054353076372  DataLoggingVariableName=ScopeData10
  StorageScope : Scope
      settings: ActiveDisplayYMinimum=-61.668067401009004  ActiveDisplayYMaximum=64.1261856723817  DataLoggingVariableName=ScopeData2
  Sum : Sum  Inputs=|+++
  TargetFloorSelector : MATLAB Function  TreatAsAtomicUnit=on
  TargetPackageFinder : MATLAB Function  TreatAsAtomicUnit=on
  Unit Delay : UnitDelay  InitialCondition=0.05  SampleTime=-1
  Unit Delay1 : UnitDelay  InitialCondition=0.20  SampleTime=-1
  Unit Delay{3..5,8..16,18} (13 alike) : UnitDelay  SampleTime=-1
  Unit Delay2 : UnitDelay  InitialCondition=0.10  SampleTime=-1
  Unit Delay6 : UnitDelay  InitialCondition=1  SampleTime=-1
  Unit Delay7 : UnitDelay  SampleTime=0.05
  UnloadController : Stateflow chart  TreatAsAtomicUnit=on  SystemSampleTime=0.05
  UnloadPrepositionFunction : MATLAB Function  TreatAsAtomicUnit=on  SystemSampleTime=0.05
  UnloadTargetManager : MATLAB Function  TreatAsAtomicUnit=on  SystemSampleTime=0.05
  VisualizationPacketFunction : MATLAB Function  TreatAsAtomicUnit=on
  floor1_count : Display
  floor1_queue : Display
  floor1_slot_id_display : Display
  floor1_used_length_display : Display
  floor2_color_flag_display : Display
  floor2_count : Display
  floor2_queue : Display
  floor2_slot_id_display : Display
  floor2_used_length_display : Display
  floor2_visible_display : Display
  floor2_x_display : Display
  floor2_y_display : Display
  floor2_yaw_display : Display
  floor2_z_display : Display
  floor3_count : Display
  floor3_queue : Display
  floor3_slot_id_display : Display
  floor3_used_length_display : Display
  floor_capacity_length : Constant
  load_target_count : Constant  Value=10
  load_target_count_display : Display
  loading_enable_display : Display
  mission_phase_display : Display
  push_count_display : Display
  state_id_display : Display
  target_count : Constant  Value=4
  target_found : Display
  target_list : Constant  Value=[3; 7; 5; 9; 0; 0; 0; 0; 0; 0; 0; 0; 0; 0; 0; 0; 0; 0; 0; 0]
  target_package_index : Display
  target_package_length : Display
  target_unload_floor : Display
  unload_state_id_display : Display
  wires:
  MainController/1(lift_cmd) -> CommandMuxFunction/2(load_lift_cmd)  "lift_cmd"
  MainController/2(target_z) -> CommandMuxFunction/3(load_target_z)  "target_z"
  MainController/6(rotator_cmd) -> RotatorControlFunction/1(rotator_cmd)  "rotator"
  MainController/7(pusher_cmd) -> PusherControlFunction/1(pusher_cmd)  "pusher"
  MainController/8(stopper_cmd) -> Mux9/3  "stopper"
  MainController/9(floor1_conv_cmd) -> CommandMuxFunction/4(load_floor1_conv_cmd)  "floor1"
  MainController/10(floor2_conv_cmd) -> CommandMuxFunction/5(load_floor2_conv_cmd)  "floor2"
  MainController/11(floor3_conv_cmd) -> CommandMuxFunction/6(load_floor3_conv_cmd)  "floor3"
  BoxSizeFunction/2(box_length) -> BoxRotationFunction/1(box_length), Mux2/2  "box_length"
  BoxSizeFunction/3(box_width) -> BoxRotationFunction/2(box_width), Mux2/3  "box_width"
  BoxRotationFunction/1(box_insert_length) -> Mux2/5, Mux17/9, TargetFloorSelector/1(box_insert_length), FloorStorageUpdate/3(box_insert_length)  "box_insert_length"
  floor_capacity_length/1 -> TargetFloorSelector/5(floor_capacity_length)
  TargetFloorSelector/1(target_floor) -> Mux6/7, MainController/1(target_floor), FloorStorageUpdate/2(target_floor), MovingPackage3DMappingFunction/11(target_floor), MATLAB Function3/3(current_target_floor), Mux17/3, Mux2/7  "target_floor_selector_out"
  Mux2/1 -> StorageScope/1
  BoxSizeFunction/1(box_type) -> Mux2/1  "box_type"
  BoxRotationFunction/2(desired_box_yaw) -> Mux2/6  "target_yaw"
  TargetFloorSelector/2(storage_available) -> MainController/3(storage_available), Mux2/8  "storage_available"
  TargetFloorSelector/3(floor1_remaining_length) -> Mux2/9, Mux17/7
  TargetFloorSelector/4(floor2_remaining_length) -> Mux17/8, Mux2/10  "floor2_remaining_length"
  TargetFloorSelector/5(floor3_remaining_length) -> Mux2/11  "floor3_remaining_length"
  MainController/12(load_done) -> FloorStorageUpdate/1(load_done), MovingPackage3DMappingFunction/8(load_done), Delay_load_done_for_box/1, Mux17/1, Unit Delay10/1, Mux3/4  "load_done"
  Unit Delay/1 -> Mux3/1, TargetFloorSelector/4(floor3_used_length), floor3_used_length_display/1  "floor3_used_length"
  FloorStorageUpdate/3(floor3_used_length) -> Unit Delay/1
  FloorStorageUpdate/2(floor2_used_length) -> Mux17/6, Unit Delay1/1
  Unit Delay1/1 -> TargetFloorSelector/3(floor2_used_length), floor2_used_length_display/1, Mux3/2  "floor2_used_length"
  FloorStorageUpdate/1(floor1_used_length) -> Mux17/5, Unit Delay2/1
  Unit Delay2/1 -> floor1_used_length_display/1, TargetFloorSelector/2(floor1_used_length), Mux3/3  "floor1_used_length"
  BoxSizeFunction/5(package_count) -> FloorStorageUpdate/4(package_id), Mux2/4  "package_count"
  BoxSizeFunction/4(box_height) -> Mux2/12  "box_height"
  Delay_load_done_for_box/1 -> BoxSizeFunction/1(load_done)
  FloorStorageUpdate/4(floor1_count) -> Mux6/1, floor1_count/1, Unit Delay3/1
  FloorStorageUpdate/5(floor2_count) -> Mux6/2, floor2_count/1, Unit Delay4/1
  FloorStorageUpdate/6(floor3_count) -> Mux6/3, floor3_count/1, Unit Delay5/1
  FloorStorageUpdate/7(floor1_queue) -> Floor1VisualStateFunction/1(floor1_queue), Mux6/4, Mux4/9, PackageSlotVisualizer/1(floor1_queue), floor1_queue/1, Delay_floor1_queue/1
  FloorStorageUpdate/8(floor2_queue) -> Floor2VisualStateFunction/1(floor2_queue), Mux4/10, floor2_queue/1, Delay_floor2_queue/1, Mux6/5, PackageSlotVisualizer/2(floor2_queue)
  FloorStorageUpdate/9(floor3_queue) -> Floor3VisualStateFunction/1(floor3_queue), PackageSlotVisualizer/3(floor3_queue), Mux7/4, Mux6/6, floor3_queue/1, Delay_floor3_queue/1
  TargetPackageFinder/3(target_package_index) -> Mux/11, Mux4/7, target_package_index/1, UnloadPrepositionFunction/5(target_package_index)
  TargetPackageFinder/2(target_unload_floor) -> CurrentUnloadReadySelector/1(target_unload_floor), Mux/10, UnloadPrepositionFunction/4(target_unload_floor), FloorStorageUpdate/7(target_unload_floor), Mux17/4, CommandMuxFunction/12(target_unload_floor), UnloadController/2(target_unload_floor), target_unload_floor/1, Mux4/6
  TargetPackageFinder/1(target_found) -> Mux4/5, UnloadPrepositionFunction/3(target_found), target_found/1
  Sum/1 -> MultiFloorUnloadPrepositionFunction/2(vehicle_stopped), Mux/2, UnloadPrepositionFunction/2(vehicle_stopped)  "vehicle_stopped"
  UnloadPrepositionFunction/3(target_package_on_belt4) -> Mux/6, Mux4/12
  UnloadController/1(unload_lift_cmd) -> Mux1/2, CommandMuxFunction/10(unload_lift_cmd)
  UnloadController/2(unload_target_z) -> Mux1/1, CommandMuxFunction/11(unload_target_z)
  UnloadController/4(belt4_reverse_cmd) -> Floor3VisualStateFunction/8(belt4_reverse_cmd), Floor1VisualStateFunction/8(belt4_reverse_cmd), Floor2VisualStateFunction/8(belt4_reverse_cmd), CommandMuxFunction/13(belt4_reverse_cmd)
  UnloadController/5(belt4_restore_cmd) -> Floor3VisualStateFunction/9(belt4_restore_cmd), Floor2VisualStateFunction/9(belt4_restore_cmd), CommandMuxFunction/14(belt4_restore_cmd), Floor1VisualStateFunction/9(belt4_restore_cmd)
  UnloadController/7(unload_done) -> Floor3VisualStateFunction/7(unload_done), Floor1VisualStateFunction/7(unload_done), Mux5/14, Delay_unload_done_to_target_manager/1, Mux4/8, FloorStorageUpdate/5(unload_done), Floor2VisualStateFunction/7(unload_done)
  Step/1 -> PlatformFoldControlFunction/2(delivery_arrived), Mux/3, UnloadController/4(delivery_arrived), MultiFloorUnloadPrepositionFunction/3(delivery_arrived)
  Mux3/1 -> Scope/1
  Delay_floor1_queue/1 -> FloorUnloadTargetSelector/3(floor1_queue), TargetPackageFinder/2(floor1_queue)
  Delay_floor2_queue/1 -> FloorUnloadTargetSelector/4(floor2_queue), TargetPackageFinder/3(floor2_queue)
  Delay_floor3_queue/1 -> FloorUnloadTargetSelector/5(floor3_queue), TargetPackageFinder/4(floor3_queue)
  FloorStorageUpdate/10(target_package_length) -> target_package_length/1
  load_target_count/1 -> MissionModeFunction/4(load_target_count), load_target_count_display/1
  MissionModeFunction/2(unload_request_auto) -> MATLAB Function1/7(highlight_enable), Package3DMappingFunction_F2/7(highlight_enable), MATLAB Function/7(highlight_enable), Unit Delay8/1
  MissionModeFunction/1(loading_enable) -> Unit Delay6/1
  Unit Delay5/1 -> MissionModeFunction/3(floor3_count)
  Unit Delay4/1 -> MissionModeFunction/2(floor2_count)
  Unit Delay3/1 -> MissionModeFunction/1(floor1_count)
  Unit Delay6/1 -> loading_enable_display/1, Mux10/2, StopperCommandFunction/2(loading_enable), MainController/4(loading_enable)  "loading_enable"
  Unit Delay8/1 -> UnloadPrepositionFunction/1(unload_request)
  MissionModeFunction/4(mission_phase) -> VisualizationPacketFunction/1(mission_phase), Mux5/2, Mux/1, MovingPackage3DMappingFunction/1(mission_phase), MultiFloorUnloadPrepositionFunction/1(mission_phase), Mux4/1, UnloadTargetManager/4(mission_phase), StopperCommandFunction/1(mission_phase), Mux10/1, mission_phase_display/1, CommandMuxFunction/1(mission_phase), PlatformFoldControlFunction/1(mission_phase), Sim3DMappingFunction/6(mission_phase)
  CommandMuxFunction/1(final_lift_cmd) -> Mux1/4, Mux5/5, Unit Delay9/1, VisualizationPacketFunction/8(final_lift_cmd)
  CommandMuxFunction/3(final_floor1_conv_cmd) -> Mux5/7, VisualizationPacketFunction/9(final_floor1_conv_cmd)
  CommandMuxFunction/4(final_floor2_conv_cmd) -> Mux5/8, VisualizationPacketFunction/10(final_floor2_conv_cmd)
  CommandMuxFunction/5(final_floor3_conv_cmd) -> Mux5/9, VisualizationPacketFunction/11(final_floor3_conv_cmd)
  CommandMuxFunction/6(final_floor1_belt4_cmd) -> Mux5/10, VisualizationPacketFunction/12(final_floor1_belt4_cmd)
  CommandMuxFunction/7(final_floor2_belt4_cmd) -> VisualizationPacketFunction/13(final_floor2_belt4_cmd), Mux5/11
  CommandMuxFunction/8(final_floor3_belt4_cmd) -> VisualizationPacketFunction/14(final_floor3_belt4_cmd), Mux5/12
  MainController/3(state_id) -> state_id_display/1, VisualizationPacketFunction/2(state_id), MovingPackage3DMappingFunction/2(state_id)  "state_id"
  UnloadController/3(unload_state_id) -> Mux1/3, Unit Delay7/1, Mux5/13, unload_state_id_display/1, VisualizationPacketFunction/3(unload_state_id)
  Unit Delay9/1 -> Gain/1
  Unit Delay10/1 -> BoxPoseFunction/1(load_done)
  BoxPoseFunction/1(box_yaw) -> MovingPackage3DMappingFunction/7(box_yaw), BoxRotationFunction/3(box_yaw)
  RotatorControlFunction/1(rotator_vel) -> Integrator/1
  Integrator/1 -> Saturation/1
  Saturation/1 -> Sim3DMappingFunction/2(rotator_angle), VisualizationPacketFunction/5(rotator_angle), RotatorControlFunction/3(rotator_angle)
  BoxRotationFunction/3(rotator_target_angle) -> RotatorControlFunction/2(rotator_target_angle)
  RotatorControlFunction/2(rotation_done) -> MovingPackage3DMappingFunction/9(rotation_done), Unit Delay11/1
  Unit Delay11/1 -> MainController/5(rotation_done)
  RotatorControlFunction/3(rotator_home_done) -> Unit Delay12/1
  Unit Delay12/1 -> MainController/6(rotator_home_done)
  PusherControlFunction/1(pusher_vel) -> Integrator2/1
  Integrator2/1 -> Saturation2/1
  Saturation2/1 -> MovingPackage3DMappingFunction/5(pusher_pos), Sim3DMappingFunction/3(pusher_pos), VisualizationPacketFunction/6(pusher_pos), PusherControlFunction/2(pusher_pos)  "pusher_pos"
  PusherControlFunction/2(push_done) -> Unit Delay13/1
  Unit Delay13/1 -> MainController/7(push_done)
  PusherControlFunction/4(push_count) -> push_count_display/1
  PusherControlFunction/3(pusher_home_done) -> Unit Delay14/1
  Unit Delay14/1 -> MainController/8(pusher_home_done)
  StopperControlFunction/1(stopper_vel) -> Integrator3/1
  Integrator3/1 -> Saturation3/1
  Saturation3/1 -> Sim3DMappingFunction/4(stopper_pos), VisualizationPacketFunction/7(stopper_pos), StopperControlFunction/2(stopper_pos)  "stopper_pos"
  StopperControlFunction/2(stopper_down_done) -> Unit Delay15/1, Mux9/1
  StopperControlFunction/3(stopper_up_done) -> Unit Delay16/1, Mux9/2
  Unit Delay15/1 -> MainController/9(stopper_down_done)
  Mux9/1 -> StopperScope/1
  StopperCommandFunction/1(stopper_cmd_final) -> StopperControlFunction/1(stopper_cmd), Mux10/3  "stopper_cmd_final"
  Mux10/1 -> StopperScopeFinal/1
  PackageSlotVisualizer/1(floor1_slot_id) -> Scope10/1, floor1_slot_id_display/1, PackageSlotToXYZFunction/1(floor1_slot_id)
  PackageSlotVisualizer/2(floor2_slot_id) -> Scope11/1, Mux/12, floor2_slot_id_display/1, PackageSlotToXYZFunction/2(floor2_slot_id)
  PackageSlotVisualizer/3(floor3_slot_id) -> Scope12/1, Mux7/3, floor3_slot_id_display/1, PackageSlotToXYZFunction/3(floor3_slot_id)
  PackageSlotToXYZFunction/3(floor2_visible) -> Package3DMappingFunction_F2/2(floor2_visible), VisualizationPacketFunction/25(floor2_visible), floor2_visible_display/1
  PackageSlotToXYZFunction/4(floor2_color_flag) -> Package3DMappingFunction_F2/3(floor2_color_flag), floor2_color_flag_display/1, VisualizationPacketFunction/26(floor2_color_flag)
  PackageSlotToXYZFunction/1(floor1_visible) -> VisualizationPacketFunction/19(floor1_visible), MATLAB Function/2(floor1_visible)
  PackageSlotToXYZFunction/2(floor1_color_flag) -> MATLAB Function/3(floor1_color_flag), VisualizationPacketFunction/20(floor1_color_flag)
  PackageSlotToXYZFunction/5(floor3_visible) -> MATLAB Function1/2(floor3_visible), VisualizationPacketFunction/31(floor3_visible), Mux7/2
  PackageSlotToXYZFunction/6(floor3_color_flag) -> MATLAB Function1/3(floor3_color_flag), VisualizationPacketFunction/32(floor3_color_flag)
  Sim3DMappingFunction/4(platform_translation) -> Platform_Actor/1  "platform_translation"
  Gain/1 -> Integrator1/1
  Integrator1/1 -> Saturation1/1
  Saturation1/1 -> UnloadController/3(platform_z), VisualizationPacketFunction/4(platform_z), MainController/2(platform_z), MATLAB Function1/10(platform_z), MATLAB Function/10(platform_z), Package3DMappingFunction_F2/10(platform_z), PlatformFoldControlFunction/3(platform_z), Sim3DMappingFunction/1(platform_z), Mux1/6  "platform_z"
  Sim3DMappingFunction/5(platform_rotation) -> Platform_Actor/2  "platform_rotation"
  Sim3DMappingFunction/6(platform_scale) -> Platform_Actor/3  "platform_scale"
  Platform_Actor/1 -> Display/1
  Sim3DMappingFunction/11(rotator_translation) -> Simulation 3D Actor/1
  Sim3DMappingFunction/12(rotator_rotation) -> Simulation 3D Actor/2
  Sim3DMappingFunction/13(rotator_scale) -> Simulation 3D Actor/3
  Simulation 3D Actor/1 -> Display1/1
  Sim3DMappingFunction/17(pusher_translation) -> Simulation 3D Actor1/1
  Sim3DMappingFunction/18(pusher_rotation) -> Simulation 3D Actor1/2
  Sim3DMappingFunction/19(pusher_scale) -> Simulation 3D Actor1/3
  Sim3DMappingFunction/23(stopper_rotation) -> Simulation 3D Actor2/2, Simulation 3D Actor4/2, Simulation 3D Actor3/2
  Sim3DMappingFunction/24(stopper_scale) -> Simulation 3D Actor2/3, Simulation 3D Actor3/3, Simulation 3D Actor4/3
  Sim3DMappingFunction/21(stopper2_translation) -> Simulation 3D Actor4/1
  Sim3DMappingFunction/22(stopper3_translation) -> Simulation 3D Actor3/1
  Sim3DMappingFunction/20(stopper1_translation) -> Simulation 3D Actor2/1
  Sim3DMappingFunction/2(platform_y) -> Package3DMappingFunction_F2/4(platform_y), Conveyor3DMappingFunction/1(platform_y), MATLAB Function1/4(platform_y), MATLAB Function/4(platform_y), MovingPackage3DMappingFunction/6(platform_y)
  Conveyor3DMappingFunction/1(belt1_f1_T) -> Belt1_F1/1
  Conveyor3DMappingFunction/2(belt2_f1_T) -> Belt2_F1/1
  Conveyor3DMappingFunction/3(belt3_f1_T) -> Belt3_F1/1
  Conveyor3DMappingFunction/4(belt4_f1_T) -> Belt4_F1/1
  Conveyor3DMappingFunction/13(belt1_S) -> Belt1_F2/3, Belt1_F1/3, Belt1_F3/3
  Conveyor3DMappingFunction/14(belt2_S) -> Belt2_F2/3, Belt2_F1/3, Belt2_F3/3
  Conveyor3DMappingFunction/15(belt3_S) -> Belt3_F2/3, Belt3_F1/3, Belt3_F3/3
  Conveyor3DMappingFunction/16(belt4_S) -> Belt4_F2/3, Belt4_F1/3, Belt4_F3/3
  Conveyor3DMappingFunction/17(belt_R) -> Belt1_F2/2, Belt4_F2/2, Belt3_F2/2, Belt2_F2/2, Belt4_F1/2, Belt3_F1/2, Belt2_F1/2, Belt1_F1/2, Belt4_F3/2, Belt3_F3/2, Belt2_F3/2, Belt1_F3/2
  Conveyor3DMappingFunction/5(belt1_f2_T) -> Belt1_F2/1
  Conveyor3DMappingFunction/6(belt2_f2_T) -> Belt2_F2/1
  Conveyor3DMappingFunction/7(belt3_f2_T) -> Belt3_F2/1
  Conveyor3DMappingFunction/8(belt4_f2_T) -> Belt4_F2/1
  Conveyor3DMappingFunction/9(belt1_f3_T) -> Belt1_F3/1
  Conveyor3DMappingFunction/10(belt2_f3_T) -> Belt2_F3/1
  Conveyor3DMappingFunction/11(belt3_f3_T) -> Belt3_F3/1
  Conveyor3DMappingFunction/12(belt4_f3_T) -> Belt4_F3/1
  Package3DMappingFunction_F2/1(pkg1_T) -> Simulation 3D Actor5/1
  Sim3DMappingFunction/3(platform_z_3d) -> MovingPackage3DMappingFunction/3(platform_z_3d)
  Sim3DMappingFunction/10(rotator_yaw) -> MovingPackage3DMappingFunction/4(rotator_yaw)
  MovingPackage3DMappingFunction/1(moving_pkg_T) -> Simulation 3D Actor10/1
  MovingPackage3DMappingFunction/2(moving_pkg_R) -> Simulation 3D Actor10/2
  MovingPackage3DMappingFunction/3(moving_pkg_S) -> Simulation 3D Actor10/3
  MovingPackage3DMappingFunction/4(moving_arrive_done) -> ArriveDoneDelayToMainController/1, MATLAB Function3/1(moving_arrive_done)
  Package3DMappingFunction_F2/2(pkg2_T) -> Simulation 3D Actor6/1
  Package3DMappingFunction_F2/3(pkg3_T) -> Simulation 3D Actor7/1
  Package3DMappingFunction_F2/4(pkg4_T) -> Simulation 3D Actor8/1
  Package3DMappingFunction_F2/5(pkg5_T) -> Simulation 3D Actor9/1
  Package3DMappingFunction_F2/6(pkg1_R) -> Simulation 3D Actor5/2
  Package3DMappingFunction_F2/7(pkg2_R) -> Simulation 3D Actor6/2
  Package3DMappingFunction_F2/8(pkg3_R) -> Simulation 3D Actor7/2
  Package3DMappingFunction_F2/9(pkg4_R) -> Simulation 3D Actor8/2
  Package3DMappingFunction_F2/10(pkg5_R) -> Simulation 3D Actor9/2
  Package3DMappingFunction_F2/11(pkg1_S) -> Simulation 3D Actor5/3
  Package3DMappingFunction_F2/12(pkg2_S) -> Simulation 3D Actor6/3
  Package3DMappingFunction_F2/13(pkg3_S) -> Simulation 3D Actor7/3
  Package3DMappingFunction_F2/14(pkg4_S) -> Simulation 3D Actor8/3
  Package3DMappingFunction_F2/15(pkg5_S) -> Simulation 3D Actor9/3
  MATLAB Function1/1(pkg1_T) -> Simulation 3D Actor14/1
  MATLAB Function1/2(pkg2_T) -> Simulation 3D Actor20/1
  MATLAB Function1/3(pkg3_T) -> Simulation 3D Actor19/1
  MATLAB Function1/4(pkg4_T) -> Simulation 3D Actor15/1
  MATLAB Function1/5(pkg5_T) -> Simulation 3D Actor16/1
  MATLAB Function1/7(pkg1_R) -> Simulation 3D Actor14/2
  MATLAB Function1/8(pkg2_R) -> Simulation 3D Actor20/2
  MATLAB Function1/9(pkg3_R) -> Simulation 3D Actor19/2
  MATLAB Function1/10(pkg4_R) -> Simulation 3D Actor15/2
  MATLAB Function1/11(pkg5_R) -> Simulation 3D Actor16/2
  MATLAB Function1/13(pkg1_S) -> Simulation 3D Actor14/3
  MATLAB Function1/14(pkg2_S) -> Simulation 3D Actor20/3
  MATLAB Function1/15(pkg3_S) -> Simulation 3D Actor19/3
  MATLAB Function1/16(pkg4_S) -> Simulation 3D Actor15/3
  MATLAB Function1/17(pkg5_S) -> Simulation 3D Actor16/3
  MATLAB Function/1(pkg1_T) -> Simulation 3D Actor11/1
  MATLAB Function/2(pkg2_T) -> Simulation 3D Actor17/1
  MATLAB Function/3(pkg3_T) -> Simulation 3D Actor18/1
  MATLAB Function/4(pkg4_T) -> Simulation 3D Actor12/1
  MATLAB Function/5(pkg5_T) -> Simulation 3D Actor13/1
  MATLAB Function/6(pkg1_R) -> Simulation 3D Actor11/2
  MATLAB Function/7(pkg2_R) -> Simulation 3D Actor17/2
  MATLAB Function/8(pkg3_R) -> Simulation 3D Actor18/2
  MATLAB Function/9(pkg4_R) -> Simulation 3D Actor12/2
  MATLAB Function/10(pkg5_R) -> Simulation 3D Actor13/2
  MATLAB Function/11(pkg1_S) -> Simulation 3D Actor11/3
  MATLAB Function/12(pkg2_S) -> Simulation 3D Actor17/3
  MATLAB Function/13(pkg3_S) -> Simulation 3D Actor18/3
  MATLAB Function/14(pkg4_S) -> Simulation 3D Actor12/3
  MATLAB Function/15(pkg5_S) -> Simulation 3D Actor13/3
  MovingPackage3DMappingFunction/5(moving_arrive_floor) -> MATLAB Function3/2(moving_arrive_floor)
  MATLAB Function3/3(visual_count_f3) -> Mux7/1
  MATLAB Function3/4(visual_count_selected) -> Unit Delay18/1
  Unit Delay18/1 -> MovingPackage3DMappingFunction/10(visual_count)
  Package3DMappingFunction_F2/16(pkg6_T) -> Simulation 3D Actor21/1
  Package3DMappingFunction_F2/17(pkg6_R) -> Simulation 3D Actor21/2
  Package3DMappingFunction_F2/18(pkg6_S) -> Simulation 3D Actor21/3
  Mux17/1 -> Scope6/1
  ArriveDoneDelayToMainController/1 -> MainController/10(moving_arrive_done)
  UnloadPrepositionFunction/1(preposition_active) -> Mux/4, Mux4/13
  UnloadPrepositionFunction/2(sensor_count) -> Mux/5, Mux4/11
  Mux/1 -> Scope2/1
  Mux1/1 -> Scope3/1
  target_count/1 -> UnloadTargetManager/2(target_count), FloorUnloadTargetSelector/2(target_count), MATLAB Function1/14(target_count), Package3DMappingFunction_F2/14(target_count), MATLAB Function/14(target_count)
  target_list/1 -> MATLAB Function/13(target_list), Package3DMappingFunction_F2/13(target_list), MATLAB Function1/13(target_list), FloorUnloadTargetSelector/1(target_list), UnloadTargetManager/1(target_list)
  UnloadTargetManager/1(target_package_id) -> Delay_current_target_package_id/1
  UnloadTargetManager/3(unload_all_done) -> Mux5/4, Mux4/4, Delay_unload_all_done_to_mission/1
  Mux4/1 -> Scope4/1
  UnloadTargetManager/2(current_target_index) -> Mux5/3, Mux4/3
  Delay_current_target_package_id/1 -> Floor3VisualStateFunction/5(current_unload_id), Floor1VisualStateFunction/5(current_unload_id), Floor2VisualStateFunction/5(current_unload_id), Mux4/2, MATLAB Function/11(current_unload_id), Package3DMappingFunction_F2/11(current_unload_id), MATLAB Function1/11(current_unload_id), Mux5/1, TargetPackageFinder/1(target_package_id), FloorStorageUpdate/6(target_package_id)
  Delay_unload_done_to_target_manager/1 -> UnloadTargetManager/3(unload_done)
  Delay_unload_all_done_to_mission/1 -> MissionModeFunction/5(unload_done)
  CommandMuxFunction/2(final_target_z) -> Mux1/5, Mux5/6
  Mux5/1 -> Scope5/1
  Mux6/1 -> Scope7/1
  Mux7/1 -> Scope8/1
  UnloadController/6(package_on_platform_from_floor) -> Floor3VisualStateFunction/6(package_on_platform_from_floor), Floor1VisualStateFunction/6(package_on_platform_from_floor), MATLAB Function/9(package_on_platform_from_floor), MATLAB Function1/9(package_on_platform_from_floor), Package3DMappingFunction_F2/9(package_on_platform_from_floor), Floor2VisualStateFunction/6(package_on_platform_from_floor)
  Step3/1 -> Sum/3
  Step2/1 -> Sum/2
  Step1/1 -> Sum/1
  UnloadPrepositionFunction/4(unload_floor1_conv_cmd) -> Mux/7
  UnloadPrepositionFunction/5(unload_floor2_conv_cmd) -> Mux/8
  UnloadPrepositionFunction/6(unload_floor3_conv_cmd) -> Mux/9
  PlatformFoldControlFunction/1(platform_fold_angle) -> Sim3DMappingFunction/5(platform_fold_angle)
  PlatformFoldControlFunction/2(platform_deployed) -> UnloadController/5(platform_deployed)
  FloorUnloadTargetSelector/1(target_id_f1) -> Floor1VisualStateFunction/3(target_id_f1), MATLAB Function/6(target_unload_id), PackageSlotToXYZFunction/4(target_id_f1), MultiFloorUnloadPrepositionFunction/6(target_id_f1)
  FloorUnloadTargetSelector/2(target_index_f1) -> MultiFloorUnloadPrepositionFunction/4(target_index_f1)
  FloorUnloadTargetSelector/3(found_f1) -> MultiFloorUnloadPrepositionFunction/5(found_f1)
  FloorUnloadTargetSelector/4(target_id_f2) -> Floor2VisualStateFunction/3(target_id_f2), PackageSlotToXYZFunction/6(target_id_f2), MultiFloorUnloadPrepositionFunction/9(target_id_f2), Package3DMappingFunction_F2/6(target_unload_id)
  FloorUnloadTargetSelector/5(target_index_f2) -> MultiFloorUnloadPrepositionFunction/7(target_index_f2)
  FloorUnloadTargetSelector/6(found_f2) -> MultiFloorUnloadPrepositionFunction/8(found_f2)
  FloorUnloadTargetSelector/7(target_id_f3) -> Floor3VisualStateFunction/3(target_id_f3), PackageSlotToXYZFunction/8(target_id_f3), MATLAB Function1/6(target_unload_id), MultiFloorUnloadPrepositionFunction/12(target_id_f3)
  FloorUnloadTargetSelector/8(target_index_f3) -> MultiFloorUnloadPrepositionFunction/10(target_index_f3)
  FloorUnloadTargetSelector/9(found_f3) -> MultiFloorUnloadPrepositionFunction/11(found_f3)
  MultiFloorUnloadPrepositionFunction/1(unload_floor1_conv_cmd) -> CommandMuxFunction/7(pre_floor1_conv_cmd)
  MultiFloorUnloadPrepositionFunction/2(unload_floor2_conv_cmd) -> CommandMuxFunction/8(pre_floor2_conv_cmd)
  MultiFloorUnloadPrepositionFunction/3(unload_floor3_conv_cmd) -> CommandMuxFunction/9(pre_floor3_conv_cmd)
  MultiFloorUnloadPrepositionFunction/4(sensor_count_f1) -> PackageSlotVisualizer/4(sensor_count_f1)
  MultiFloorUnloadPrepositionFunction/5(sensor_count_f2) -> PackageSlotVisualizer/5(sensor_count_f2)
  MultiFloorUnloadPrepositionFunction/6(sensor_count_f3) -> PackageSlotVisualizer/6(sensor_count_f3)
  MultiFloorUnloadPrepositionFunction/7(target_on_belt4_f1) -> Floor1VisualStateFunction/4(target_on_belt4_f1), CurrentUnloadReadySelector/2(target_on_belt4_f1), MATLAB Function/8(target_package_on_belt4), PackageSlotToXYZFunction/5(target_on_belt4_f1)
  MultiFloorUnloadPrepositionFunction/8(target_on_belt4_f2) -> Package3DMappingFunction_F2/8(target_package_on_belt4), PackageSlotToXYZFunction/7(target_on_belt4_f2), CurrentUnloadReadySelector/3(target_on_belt4_f2), Floor2VisualStateFunction/4(target_on_belt4_f2)
  MultiFloorUnloadPrepositionFunction/9(target_on_belt4_f3) -> Floor3VisualStateFunction/4(target_on_belt4_f3), CurrentUnloadReadySelector/4(target_on_belt4_f3), MATLAB Function1/8(target_package_on_belt4), PackageSlotToXYZFunction/9(target_on_belt4_f3)
  CurrentUnloadReadySelector/1(current_target_on_belt4) -> UnloadController/1(target_package_on_belt4)
  Unit Delay7/1 -> MultiFloorUnloadPrepositionFunction/13(unload_state_id_for_preposition)
  MultiFloorUnloadPrepositionFunction/13(visual_shift_f1) -> Floor1VisualStateFunction/2(visual_shift_f1), Mux8/1
  MultiFloorUnloadPrepositionFunction/14(visual_shift_f2) -> Floor2VisualStateFunction/2(visual_shift_f2), Mux8/2
  MultiFloorUnloadPrepositionFunction/15(visual_shift_f3) -> Floor3VisualStateFunction/2(visual_shift_f3), Mux8/3
  Mux8/1 -> Scope9/1
  Package3DMappingFunction_F2/19(pkg1_Color) -> Simulation 3D Actor5/4
  Package3DMappingFunction_F2/20(pkg2_Color) -> Simulation 3D Actor6/4
  Package3DMappingFunction_F2/21(pkg3_Color) -> Simulation 3D Actor7/4
  Package3DMappingFunction_F2/22(pkg4_Color) -> Simulation 3D Actor8/4
  Package3DMappingFunction_F2/23(pkg5_Color) -> Simulation 3D Actor9/4
  Package3DMappingFunction_F2/24(pkg6_Color) -> Simulation 3D Actor21/4
  Floor2VisualStateFunction/1(floor2_visual_id) -> Package3DMappingFunction_F2/1(floor2_visual_id)
  Floor2VisualStateFunction/2(floor2_visual_path) -> Package3DMappingFunction_F2/12(floor2_visual_path)
  Floor2VisualStateFunction/3(floor2_visual_count) -> Package3DMappingFunction_F2/5(floor2_visual_count)
  Floor1VisualStateFunction/1(floor1_visual_id) -> MATLAB Function/1(floor1_visual_id)
  Floor1VisualStateFunction/3(floor1_visual_count) -> MATLAB Function/5(floor1_visual_count)
  Floor1VisualStateFunction/2(floor1_visual_path) -> MATLAB Function/12(floor1_visual_path)
  MATLAB Function/16(pkg1_Color) -> Simulation 3D Actor11/4
  MATLAB Function/17(pkg2_Color) -> Simulation 3D Actor17/4
  MATLAB Function/18(pkg3_Color) -> Simulation 3D Actor18/4
  MATLAB Function/19(pkg4_Color) -> Simulation 3D Actor12/4
  MATLAB Function/20(pkg5_Color) -> Simulation 3D Actor13/4
  Floor3VisualStateFunction/2(floor3_visual_path) -> MATLAB Function1/12(floor3_visual_path)
  Floor3VisualStateFunction/3(floor3_visual_count) -> MATLAB Function1/5(floor3_visual_count)
  Floor3VisualStateFunction/1(floor3_visual_id) -> MATLAB Function1/1(floor3_visual_id)
  MATLAB Function1/19(pkg1_Color) -> Simulation 3D Actor14/4
  MATLAB Function1/20(pkg2_Color) -> Simulation 3D Actor20/4
  MATLAB Function1/21(pkg3_Color) -> Simulation 3D Actor19/4
  MATLAB Function1/22(pkg4_Color) -> Simulation 3D Actor15/4
  MATLAB Function1/23(pkg5_Color) -> Simulation 3D Actor16/4
  Floor2VisualStateFunction/4(belt4_reverse_progress) -> Package3DMappingFunction_F2/15(belt4_reverse_progress)
  Floor2VisualStateFunction/5(belt4_reverse_phase) -> Package3DMappingFunction_F2/16(belt4_reverse_phase)
  Floor1VisualStateFunction/4(belt4_reverse_progress) -> MATLAB Function/15(belt4_reverse_progress)
  Floor1VisualStateFunction/5(belt4_reverse_phase) -> MATLAB Function/16(belt4_reverse_phase)
  Floor3VisualStateFunction/4(belt4_reverse_progress) -> MATLAB Function1/15(belt4_reverse_progress)
  Floor3VisualStateFunction/5(belt4_reverse_phase) -> MATLAB Function1/16(belt4_reverse_phase)
